simulink model "test_buildingblocks_newbasicblk_20150723"  (R2014a)
settings: Solver=ode45  StartTime=0.0  StopTime=100  FixedStep=0.001e-3  RelTol=1e-8  AbsTol=1e-11
values from neighbouring files (symbols this model uses):
  A_FB_EN = 1    [test_buildingblocks_newbasicblk_20150723_Sim.m]
  A_FB_EN0 = 1    [test_buildingblocks_newbasicblk_20150723_Sim.m]
  A_FB_EN01 = 0    [test_buildingblocks_newbasicblk_20150723_Sim.m]
  A_FB_EN1 = 1    [test_buildingblocks_newbasicblk_20150723_Sim.m]
  A_FB_EN12 = 0    [test_buildingblocks_newbasicblk_20150723_Sim.m]
  A_FB_EN4 = 0.5    [test_buildingblocks_newbasicblk_20150723_Sim.m]
  A_FB_EN5 = 0    [test_buildingblocks_newbasicblk_20150723_Sim.m]
  A_FB_EN_FI = 0    [test_buildingblocks_newbasicblk_20150723_Sim.m]
  B_FB_EN = 1    [test_buildingblocks_newbasicblk_20150723_Sim.m]
  B_FB_EN0 = 1    [test_buildingblocks_newbasicblk_20150723_Sim.m]
  B_FB_EN01 = 0    [test_buildingblocks_newbasicblk_20150723_Sim.m]
  B_FB_EN1 = 0    [test_buildingblocks_newbasicblk_20150723_Sim.m]
  B_FB_EN11 = 1    [test_buildingblocks_newbasicblk_20150723_Sim.m]
  B_FB_EN12 = 0    [test_buildingblocks_newbasicblk_20150723_Sim.m]
  B_FB_EN_FI = 0    [test_buildingblocks_newbasicblk_20150723_Sim.m]
  C_FF_EN = 1    [test_buildingblocks_newbasicblk_20150723_Sim.m]
  C_FF_ENb = 0    [test_buildingblocks_newbasicblk_20150723_Sim.m]
  D_FF_EN = 1    [test_buildingblocks_newbasicblk_20150723_Sim.m]
  D_FF_EN1 = 1    [test_buildingblocks_newbasicblk_20150723_Sim.m]
  KDfw = 10    [test_buildingblocks_newbasicblk_20150723_Model.m]    (also in test_buildingblocks_newbasicblk_20150723_Sim.m)
  KDfw0 = 10    [test_buildingblocks_newbasicblk_20150723_Sim.m]
  KDfw01 = 5    [test_buildingblocks_newbasicblk_20150723_Model.m]    (also in test_buildingblocks_newbasicblk_20150723_Sim.m)
  KDfw02 = 10    [test_buildingblocks_newbasicblk_20150723_Model.m]    (also in test_buildingblocks_newbasicblk_20150723_Sim.m)
  KDfw03 = 30    [test_buildingblocks_newbasicblk_20150723_Model.m]    (also in test_buildingblocks_newbasicblk_20150723_Sim.m)
  KDfw2 = 10    [test_buildingblocks_newbasicblk_20150723_Sim.m]
  KDrv = 10    [test_buildingblocks_newbasicblk_20150723_Model.m]    (also in test_buildingblocks_newbasicblk_20150723_Sim.m)
  KDrv0 = 10    [test_buildingblocks_newbasicblk_20150723_Sim.m]
  KDrv01 = 10    [test_buildingblocks_newbasicblk_20150723_Model.m]    (also in test_buildingblocks_newbasicblk_20150723_Sim.m)
  KDrv02 = 5    [test_buildingblocks_newbasicblk_20150723_Model.m]    (also in test_buildingblocks_newbasicblk_20150723_Sim.m)
  KDrv03 = 10    [test_buildingblocks_newbasicblk_20150723_Model.m]    (also in test_buildingblocks_newbasicblk_20150723_Sim.m)
  KDrv2 = 10    [test_buildingblocks_newbasicblk_20150723_Sim.m]
  KDrv5 = 10000000    [test_buildingblocks_newbasicblk_20150723_Sim.m]
  KDrv6 = 10000000    [test_buildingblocks_newbasicblk_20150723_Sim.m]
  kr1 = 10*kr_1/KDrv01    (= 10)    [test_buildingblocks_newbasicblk_20150723_Model.m]    (also in test_buildingblocks_newbasicblk_20150723_Sim.m)
  kr11 = 10    [test_buildingblocks_newbasicblk_20150723_Sim.m]
  kr1_01 = 5    [test_buildingblocks_newbasicblk_20150723_Sim.m]
  kr2 = 10*kr_1/KDrv02    (= 20)    [test_buildingblocks_newbasicblk_20150723_Model.m]    (also in test_buildingblocks_newbasicblk_20150723_Sim.m = 5)
  kr22 = 5    [test_buildingblocks_newbasicblk_20150723_Sim.m]
  krC = 10    [test_buildingblocks_newbasicblk_20150723_Sim.m]
  krC4 = 20    [test_buildingblocks_newbasicblk_20150723_Sim.m]
  krD = 10    [test_buildingblocks_newbasicblk_20150723_Sim.m]
  n = 1    [test_buildingblocks_newbasicblk_20150723_Sim.m]
  ratC = 0    [test_buildingblocks_newbasicblk_20150723_Sim.m]
  ratC0 = 0    [test_buildingblocks_newbasicblk_20150723_Sim.m]
  ratC01 = 1    [test_buildingblocks_newbasicblk_20150723_Sim.m]
  ratC02 = 0.1    [test_buildingblocks_newbasicblk_20150723_Sim.m]
  ratC03 = 2    [test_buildingblocks_newbasicblk_20150723_Sim.m]
  ratC04 = 0.5    [test_buildingblocks_newbasicblk_20150723_Sim.m]
  ratC05 = 10    [test_buildingblocks_newbasicblk_20150723_Sim.m]
  ratC10 = 0.06    [test_buildingblocks_newbasicblk_20150723_Model.m]    (also in test_buildingblocks_newbasicblk_20150723_Sim.m = 0.6)
  ratC11 = 0.2    [test_buildingblocks_newbasicblk_20150723_Sim.m]
  ratC12 = 0.2    [test_buildingblocks_newbasicblk_20150723_Model.m]    (also in test_buildingblocks_newbasicblk_20150723_Sim.m = 1)
  ratC13 = 0.2    [test_buildingblocks_newbasicblk_20150723_Model.m]    (also in test_buildingblocks_newbasicblk_20150723_Sim.m = 2)
  ratC14 = 0.3    [test_buildingblocks_newbasicblk_20150723_Model.m]    (also in test_buildingblocks_newbasicblk_20150723_Sim.m = 3)
  ratC15 = 0.2    [test_buildingblocks_newbasicblk_20150723_Model.m]    (also in test_buildingblocks_newbasicblk_20150723_Sim.m = 10)
  ratC4 = 1    [test_buildingblocks_newbasicblk_20150723_Model.m]    (also in test_buildingblocks_newbasicblk_20150723_Sim.m)
  ratC5 = 3    [test_buildingblocks_newbasicblk_20150723_Model.m]    (also in test_buildingblocks_newbasicblk_20150723_Sim.m)
  ratC7 = 1    [test_buildingblocks_newbasicblk_20150723_Model.m]    (also in test_buildingblocks_newbasicblk_20150723_Sim.m = 2)
  ratC8 = 0.1    [test_buildingblocks_newbasicblk_20150723_Model.m]    (also in test_buildingblocks_newbasicblk_20150723_Sim.m)
  ratC9 = 0.03    [test_buildingblocks_newbasicblk_20150723_Model.m]    (also in test_buildingblocks_newbasicblk_20150723_Sim.m = 0)
  ratD = 0    [test_buildingblocks_newbasicblk_20150723_Sim.m]
(part 1 of 3)
settings Model: Creator=lorenzo  LastModifiedBy=Sung
settings SolverCC: ZeroCrossControl=DisableAll
settings DataIOCC: SignalLoggingSaveFormat=ModelDataLogs
settings OptimizationCC: ExpressionDepthLimit=2147483647
settings DebuggingCC: UnderspecifiedInitializationDetection=Classic  FcnCallInpInsideContextMsg=UseLocalSettings  StateNameClashWarn=warning
settings GRTTargetCC: CombineOutputUpdateFcns=off  GRTInterface=on

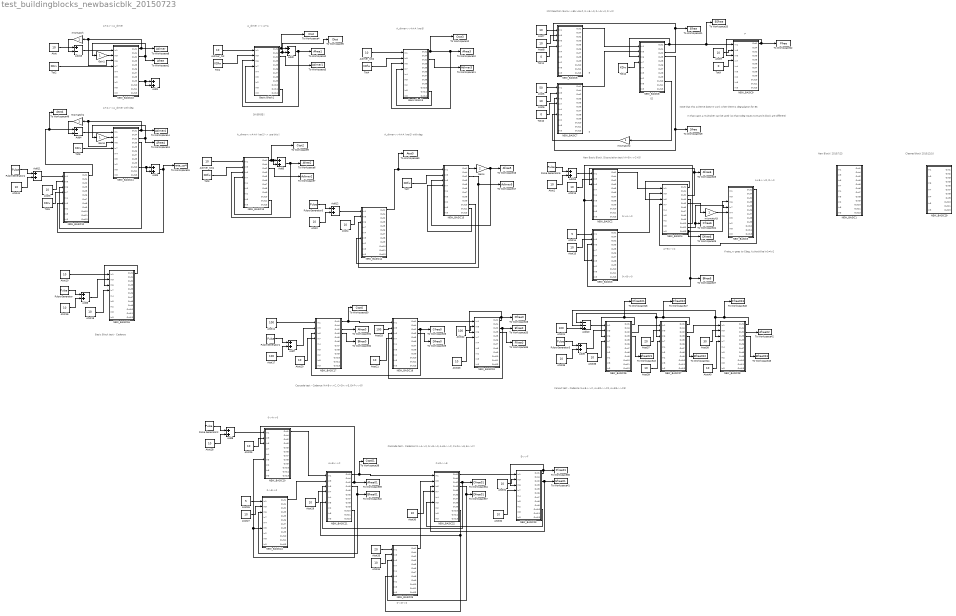
== system test_buildingblocks_newbasicblk_20150723 ==
  note: A+A<->A_dimer
  note: A_dimer <-> A+A
  note: DIVERGE!!
  note: A_dimer<->A+A (ver2) -> use this!!
  note: A_dimer<->A+A (ver3)
  note: A+A<->A_dimer with deg
  note: A_dimer<->A+A (ver2) with deg
  note: MM Reaction (E+S<->ES->E+P, 0->E->0, 0->S->0, P->0)
  note: P
  note: E
  note: S
  note: ES
  note: New Basic Block. Dissociation test (A+B<->C+D)
  note: A+B<->D, D->0
  note: A+B<->C
  note: 0->A->0
  note: 0->B->0
  note: New Block! 2015/7/23
  note: If rate_rv goes to Cdeg, it should be kr1=kr2
  note: Note that this scheme doesn't work when there is degradation for ES
  note: In that case, a multiplier can be used (so that Cdeg inputs to E and S block are different)
  note: Basic Block test - Cadence
  note: Cascade test - Cadence (A+B<->C, C+D<->E, E+F<->G)
  note: Cascade test - Cadence (0->A->0, 0->B->0, A+B<->C, C+D<->E, E<->F)
  note: 0->A->0
  note: A+B<->C
  note: 0->B->0
  note: C+D<->E
  note: E<->F
  note: 0->D->0
  note: Fanout test - Cadence (A+B<->C, A+B2<->C2, A+B3<->C3)
  note: Cleaned block 2015/12/10
  Add{1..3,5..9,11..13} (11 alike) : Sum
  Add10 : Sum  Inputs=--+
  Add15 : Sum  Inputs=+-
  Add4 : Sum  Inputs=+-
  Adimer_tot : Constant  Value=10
  Adimer_tot1 : Constant  Value=10
  Adimer_tot2 : Constant  Value=10
  Atot{,1..4,6..10,13,15..16,19..21,23,25,27..32,34..36,39..41} (30 alike) : Constant  Value=10
  Atot{11,17..18,22,24} (5 alike) : Constant  Value=100
  Atot14 : Constant  Value=5
  Atot26 : Constant  Value=5
  Atot33 : Constant  Value=20
  Atot37 : Constant  Value=20
  Atot38 : Constant  Value=30
  Atot5 : Constant  Value=50
  Basic Block1 : Subsystem
  Basic Block3 : Subsystem
  Gain1 : Gain
  Gain3 : Gain
  Gain4 : Gain  Gain=2
  NEW_BASIC1 : Subsystem
  NEW_BASIC10 : Subsystem
  NEW_BASIC11 : Subsystem
  NEW_BASIC12 : Subsystem
  NEW_BASIC13 : Subsystem
  NEW_BASIC14 : Subsystem
  NEW_BASIC15 : Subsystem
  NEW_BASIC16 : Subsystem
  NEW_BASIC17 : Subsystem
  NEW_BASIC18 : Subsystem
  NEW_BASIC19 : Subsystem
  NEW_BASIC2 : Subsystem
  NEW_BASIC20 : Subsystem
  NEW_BASIC21 : Subsystem
  NEW_BASIC22 : Subsystem
  NEW_BASIC23 : Subsystem
  NEW_BASIC24 : Subsystem
  NEW_BASIC25 : Subsystem
  NEW_BASIC26 : Subsystem
  NEW_BASIC27 : Subsystem
  NEW_BASIC28 : Subsystem
  NEW_BASIC29 : Subsystem
  NEW_BASIC3 : Subsystem
  NEW_BASIC4 : Subsystem
  NEW_BASIC5 : Subsystem
  NEW_BASIC6 : Subsystem
  NEW_BASIC7 : Subsystem
  NEW_BASIC8 : Subsystem
  NEW_BASIC9 : Subsystem
  Pulse Generator{,2..3,6} (4 alike) : DiscretePulseGenerator  PulseType=Time based  Amplitude=10  PulseWidth=50
  Pulse Generator1 : DiscretePulseGenerator  PulseType=Time based  Amplitude=100  PulseWidth=50
  Pulse Generator4 : DiscretePulseGenerator  PulseType=Time based  Amplitude=10  Period=4  PulseWidth=50
  Pulse Generator5 : DiscretePulseGenerator  PulseType=Time based  Amplitude=10  Period=4  PulseWidth=50
  To Workspace1 : ToWorkspace  VariableName=Afree  SaveFormat=Timeseries  SampleTime=-1
  To Workspace10 : ToWorkspace  VariableName=Afree3  SaveFormat=Timeseries  SampleTime=-1
  To Workspace11 : ToWorkspace  VariableName=Adimer3  SaveFormat=Timeseries  SampleTime=-1
  To Workspace12 : ToWorkspace  VariableName=Ctot3  SaveFormat=Timeseries  SampleTime=-1
  To Workspace13 : ToWorkspace  VariableName=Afree4  SaveFormat=Timeseries  SampleTime=-1
  To Workspace14 : ToWorkspace  VariableName=Adimer4  SaveFormat=Timeseries  SampleTime=-1
  To Workspace15 : ToWorkspace  VariableName=rate_up4  SaveFormat=Timeseries  SampleTime=-1
  To Workspace16 : ToWorkspace  VariableName=Afree5  SaveFormat=Timeseries  SampleTime=-1
  To Workspace17 : ToWorkspace  VariableName=Adimer5  SaveFormat=Timeseries  SampleTime=-1
  To Workspace19 : ToWorkspace  VariableName=Sfree  SaveFormat=Timeseries  SampleTime=-1
  To Workspace2 : ToWorkspace  VariableName=Afree1  SaveFormat=Timeseries  SampleTime=-1
  To Workspace20 : ToWorkspace  VariableName=ESfree  SaveFormat=Timeseries  SampleTime=-1
  To Workspace21 : ToWorkspace  VariableName=Efree  SaveFormat=Timeseries  SampleTime=-1
  To Workspace22 : ToWorkspace  VariableName=Pfree  SaveFormat=Timeseries  SampleTime=-1
  To Workspace23 : ToWorkspace  VariableName=Afree6  SaveFormat=Timeseries  SampleTime=-1
  To Workspace24 : ToWorkspace  VariableName=Cfree6  SaveFormat=Timeseries  SampleTime=-1
  To Workspace25 : ToWorkspace  VariableName=Dfree6  SaveFormat=Timeseries  SampleTime=-1
  To Workspace26 : ToWorkspace  VariableName=Cfree0  SaveFormat=Timeseries  SampleTime=-1
  To Workspace27 : ToWorkspace  VariableName=Bfree6  SaveFormat=Timeseries  SampleTime=-1
  To Workspace28 : ToWorkspace  VariableName=Gfree0  SaveFormat=Timeseries  SampleTime=-1
  To Workspace29 : ToWorkspace  VariableName=Dfree0  SaveFormat=Timeseries  SampleTime=-1
  To Workspace3 : ToWorkspace  VariableName=Adimer1  SaveFormat=Timeseries  SampleTime=-1
  To Workspace30 : ToWorkspace  VariableName=Ctot0  SaveFormat=Timeseries  SampleTime=-1
  To Workspace31 : ToWorkspace  VariableName=Afree0  SaveFormat=Timeseries  SampleTime=-1
  To Workspace32 : ToWorkspace  VariableName=Bfree0  SaveFormat=Timeseries  SampleTime=-1
  To Workspace33 : ToWorkspace  VariableName=Efree0  SaveFormat=Timeseries  SampleTime=-1
  To Workspace34 : ToWorkspace  VariableName=Cfree01  SaveFormat=Timeseries  SampleTime=-1
  To Workspace35 : ToWorkspace  VariableName=Ffree0  SaveFormat=Timeseries  SampleTime=-1
  To Workspace36 : ToWorkspace  VariableName=Ffree01  SaveFormat=Timeseries  SampleTime=-1
  To Workspace37 : ToWorkspace  VariableName=Dfree01  SaveFormat=Timeseries  SampleTime=-1
  To Workspace38 : ToWorkspace  VariableName=Ctot01  SaveFormat=Timeseries  SampleTime=-1
  To Workspace39 : ToWorkspace  VariableName=Afree01  SaveFormat=Timeseries  SampleTime=-1
  To Workspace4 : ToWorkspace  VariableName=Ctot  SaveFormat=Timeseries  SampleTime=-1
  To Workspace40 : ToWorkspace  VariableName=Bfree01  SaveFormat=Timeseries  SampleTime=-1
  To Workspace41 : ToWorkspace  VariableName=Efree01  SaveFormat=Timeseries  SampleTime=-1
  To Workspace42 : ToWorkspace  VariableName=Afree02  SaveFormat=Timeseries  SampleTime=-1
  To Workspace43 : ToWorkspace  VariableName=Bfree021  SaveFormat=Timeseries  SampleTime=-1
  To Workspace44 : ToWorkspace  VariableName=Bfree022  SaveFormat=Timeseries  SampleTime=-1
  To Workspace45 : ToWorkspace  VariableName=Bfree023  SaveFormat=Timeseries  SampleTime=-1
  To Workspace46 : ToWorkspace  VariableName=Cfree021  SaveFormat=Timeseries  SampleTime=-1
  To Workspace47 : ToWorkspace  VariableName=Cfree022  SaveFormat=Timeseries  SampleTime=-1
  To Workspace48 : ToWorkspace  VariableName=Cfree023  SaveFormat=Timeseries  SampleTime=-1
  To Workspace49 : ToWorkspace  VariableName=Atot4  SaveFormat=Timeseries  SampleTime=-1
  To Workspace5 : ToWorkspace  VariableName=Dtot  SaveFormat=Timeseries  SampleTime=-1
  To Workspace50 : ToWorkspace  VariableName=Atot5  SaveFormat=Timeseries  SampleTime=-1
  To Workspace6 : ToWorkspace  VariableName=Afree2  SaveFormat=Timeseries  SampleTime=-1
  To Workspace7 : ToWorkspace  VariableName=Adimer2  SaveFormat=Timeseries  SampleTime=-1
  To Workspace8 : ToWorkspace  VariableName=Adimer  SaveFormat=Timeseries  SampleTime=-1
  To Workspace9 : ToWorkspace  VariableName=Ctot2  SaveFormat=Timeseries  SampleTime=-1
  Tot{1,3..4,7} (4 alike) : Constant  Value=KDfw
  Tot10 : Constant  Value=0
  Tot11 : Constant  Value=0
  Tot{2,5..6,12} (4 alike) : Constant  Value=KDrv
  Tot9 : Constant  Value=0
  mismatch{,1..3} (4 alike) : Gain
  wires:
  Add15/1 -> NEW_BASIC10/1(In1)
  Atot/1 -> Add15/1
  NEW_BASIC10/1(Out1) -> To Workspace8/1, NEW_BASIC10/3(In6), mismatch/1
  NEW_BASIC10/3(Out2) -> To Workspace1/1, Gain1/1
  Tot2/1 -> NEW_BASIC10/4(In7)
  Adimer_tot/1 -> Basic Block1/1(In1)
  Basic Block1/11(Out11) -> Basic Block1/4(In7)
  Tot1/1 -> Basic Block1/2(In9)
  Basic Block1/1(Out1) -> To Workspace4/1, Add2/1
  Basic Block1/2(Out4) -> To Workspace5/1, Add2/2
  Add2/1 -> To Workspace2/1, Basic Block1/3(In6)
  Basic Block1/3(Out2) -> To Workspace3/1
  Adimer_tot1/1 -> NEW_BASIC13/1(In1)
  Tot3/1 -> NEW_BASIC13/2(In9)
  NEW_BASIC13/1(Out1) -> Add5/2, Add5/1, To Workspace9/1
  Add5/1 -> NEW_BASIC13/3(In6), To Workspace6/1
  NEW_BASIC13/3(Out2) -> To Workspace7/1
  NEW_BASIC13/11(Out11) -> NEW_BASIC13/4(In7)
  Adimer_tot2/1 -> Basic Block3/1(In1)
  Tot4/1 -> Basic Block3/2(In9)
  Basic Block3/1(Out1) -> Basic Block3/3(In6), To Workspace10/1, To Workspace12/1
  Basic Block3/3(Out2) -> To Workspace11/1
  Basic Block3/11(Out11) -> Basic Block3/4(In7)
  mismatch/1 -> Add15/2
  Gain1/1 -> NEW_BASIC10/2(In9)
  NEW_BASIC10/9(Out9) -> Add1/2, Add1/1
  Add4/1 -> NEW_BASIC11/1(In1)
  NEW_BASIC12/1(Out1) -> To Workspace49/1, Add4/1
  NEW_BASIC11/1(Out1) -> NEW_BASIC11/3(In6), mismatch1/1, To Workspace14/1
  NEW_BASIC11/3(Out2) -> Gain3/1, To Workspace13/1
  Tot5/1 -> NEW_BASIC11/4(In7)
  mismatch1/1 -> Add4/2
  Gain3/1 -> NEW_BASIC11/2(In9)
  Add11/1 -> NEW_BASIC12/1(In1)
  Atot3/1 -> NEW_BASIC12/2(In9)
  Tot6/1 -> NEW_BASIC12/4(In7)
  NEW_BASIC11/4(Out3) -> NEW_BASIC12/3(In6)
  Add3/1 -> NEW_BASIC12/6(In5), To Workspace15/1
  NEW_BASIC11/10(Out10) -> Add3/2, Add3/1
  NEW_BASIC14/1(Out1) -> To Workspace50/1, NEW_BASIC15/1(In1)
  Tot7/1 -> NEW_BASIC15/2(In9)
  NEW_BASIC15/1(Out1) -> Gain4/1
  Gain4/1 -> NEW_BASIC15/3(In6), To Workspace16/1
  NEW_BASIC15/3(Out2) -> NEW_BASIC14/3(In6), To Workspace17/1
  NEW_BASIC15/11(Out11) -> NEW_BASIC15/4(In7)
  Atot4/1 -> NEW_BASIC14/2(In9)
  NEW_BASIC15/10(Out10) -> NEW_BASIC14/6(In5)
  Atot5/1 -> NEW_BASIC7/1(In1)
  Atot6/1 -> NEW_BASIC7/2(In9)
  Tot10/1 -> NEW_BASIC7/4(In7)
  NEW_BASIC8/10(Out10) -> mismatch2/1
  Atot7/1 -> NEW_BASIC6/1(In1)
  Atot8/1 -> NEW_BASIC6/2(In9)
  Tot11/1 -> NEW_BASIC6/4(In7)
  NEW_BASIC6/1(Out1) -> NEW_BASIC8/1(In1)
  NEW_BASIC7/1(Out1) -> NEW_BASIC8/2(In9)
  NEW_BASIC8/3(Out2) -> NEW_BASIC6/3(In6), To Workspace21/1
  NEW_BASIC8/4(Out3) -> NEW_BASIC7/3(In6), To Workspace19/1
  NEW_BASIC8/1(Out1) -> NEW_BASIC8/3(In6), NEW_BASIC9/1(In1), To Workspace20/1
  Atot9/1 -> NEW_BASIC9/2(In9)
  Tot9/1 -> NEW_BASIC9/4(In7)
  NEW_BASIC9/1(Out1) -> NEW_BASIC9/3(In6), To Workspace22/1
  Tot12/1 -> NEW_BASIC8/4(In7)
  mismatch2/1 -> NEW_BASIC7/6(In5)
  NEW_BASIC4/5(Out5) -> mismatch3/1
  NEW_BASIC4/1(Out1) -> NEW_BASIC4/3(In6)
  NEW_BASIC5/1(Out1) -> NEW_BASIC4/4(In7)
  NEW_BASIC4/11(Out11) -> NEW_BASIC5/4(In7), To Workspace24/1
  NEW_BASIC4/12(Out13) -> NEW_BASIC5/3(In6), To Workspace25/1
  NEW_BASIC4/4(Out3) -> NEW_BASIC3/3(In6), To Workspace27/1
  mismatch3/1 -> NEW_BASIC5/5(In4)
  Atot13/1 -> NEW_BASIC2/2(In9)
  Atot14/1 -> NEW_BASIC3/1(In1)
  Atot15/1 -> NEW_BASIC3/2(In9)
  NEW_BASIC2/1(Out1) -> NEW_BASIC4/1(In1)
  NEW_BASIC3/1(Out1) -> NEW_BASIC4/2(In9)
  NEW_BASIC4/3(Out2) -> NEW_BASIC2/3(In6), To Workspace23/1
  NEW_BASIC4/10(Out10) -> NEW_BASIC3/6(In5), NEW_BASIC2/6(In5)
  Atot10/1 -> NEW_BASIC16/1(In1)
  NEW_BASIC16/1(Out1) -> NEW_BASIC16/3(In6)
  Pulse Generator/1 -> Add6/1
  Atot16/1 -> Add6/2
  Add6/1 -> NEW_BASIC16/2(In9)
  Atot11/1 -> NEW_BASIC17/1(In1)
  Pulse Generator1/1 -> Add7/1
  Atot17/1 -> Add7/2
  Add7/1 -> NEW_BASIC17/2(In9)
  NEW_BASIC17/1(Out1) -> To Workspace30/1, NEW_BASIC18/1(In1)
  Atot18/1 -> NEW_BASIC18/2(In9)
  NEW_BASIC18/3(Out2) -> To Workspace26/1, NEW_BASIC17/3(In6)
  Atot19/1 -> NEW_BASIC16/4(In7)
  Atot20/1 -> NEW_BASIC17/4(In7)
  Atot21/1 -> NEW_BASIC18/4(In7)
  NEW_BASIC17/3(Out2) -> To Workspace31/1
  NEW_BASIC17/4(Out3) -> To Workspace32/1
  NEW_BASIC18/4(Out3) -> To Workspace29/1
  Atot22/1 -> NEW_BASIC19/2(In9)
  Atot23/1 -> NEW_BASIC19/4(In7)
  NEW_BASIC19/4(Out3) -> To Workspace35/1
  NEW_BASIC18/1(Out1) -> NEW_BASIC19/1(In1)
  NEW_BASIC19/1(Out1) -> To Workspace28/1, NEW_BASIC19/3(In6)
  NEW_BASIC19/3(Out2) -> NEW_BASIC18/3(In6), To Workspace33/1
  Add8/1 -> NEW_BASIC20/1(In1)
  Atot25/1 -> NEW_BASIC20/2(In9)
  NEW_BASIC21/1(Out1) -> NEW_BASIC22/1(In1), To Workspace38/1
  NEW_BASIC22/3(Out2) -> NEW_BASIC21/3(In6), To Workspace34/1
  Atot29/1 -> NEW_BASIC21/4(In7)
  Atot30/1 -> NEW_BASIC22/4(In7)
  NEW_BASIC21/3(Out2) -> NEW_BASIC20/3(In6), To Workspace39/1
  NEW_BASIC21/4(Out3) -> NEW_BASIC24/3(In6), To Workspace40/1
  NEW_BASIC22/4(Out3) -> NEW_BASIC25/3(In6), To Workspace37/1
  Atot31/1 -> NEW_BASIC23/2(In9)
  Atot32/1 -> NEW_BASIC23/4(In7)
  NEW_BASIC22/1(Out1) -> NEW_BASIC23/1(In1)
  NEW_BASIC23/1(Out1) -> NEW_BASIC23/3(In6), To Workspace36/1
  NEW_BASIC23/3(Out2) -> To Workspace41/1, NEW_BASIC22/3(In6)
  Atot26/1 -> NEW_BASIC24/1(In1)
  Atot27/1 -> NEW_BASIC24/2(In9)
  NEW_BASIC20/1(Out1) -> NEW_BASIC21/1(In1)
  NEW_BASIC24/1(Out1) -> NEW_BASIC21/2(In9)
  Atot33/1 -> NEW_BASIC25/1(In1)
  Atot34/1 -> NEW_BASIC25/2(In9)
  NEW_BASIC25/1(Out1) -> NEW_BASIC22/2(In9)
  NEW_BASIC23/10(Out10) -> NEW_BASIC22/6(In5)
  NEW_BASIC22/10(Out10) -> NEW_BASIC25/6(In5), NEW_BASIC21/6(In5)
  NEW_BASIC21/10(Out10) -> NEW_BASIC24/6(In5), NEW_BASIC20/6(In5)
  Pulse Generator2/1 -> Add8/1
  Atot28/1 -> Add8/2
  Pulse Generator3/1 -> Add9/1
  Atot35/1 -> Add9/2
  Add9/1 -> NEW_BASIC26/2(In9)
  NEW_BASIC26/1(Out1) -> To Workspace46/1, NEW_BASIC26/3(In6)
  Add10/1 -> NEW_BASIC26/1(In1)
  Atot24/1 -> Add10/3
  NEW_BASIC27/1(Out1) -> To Workspace47/1, Add10/1, NEW_BASIC27/3(In6)
  NEW_BASIC28/1(Out1) -> To Workspace48/1, NEW_BASIC28/3(In6), Add10/2
  NEW_BASIC26/3(Out2) -> NEW_BASIC27/1(In1)
  NEW_BASIC27/3(Out2) -> NEW_BASIC28/1(In1)
  NEW_BASIC28/3(Out2) -> To Workspace42/1
  Atot37/1 -> NEW_BASIC27/2(In9)
  Atot38/1 -> NEW_BASIC28/2(In9)
  NEW_BASIC26/4(Out3) -> To Workspace43/1
  NEW_BASIC28/4(Out3) -> To Workspace45/1
  NEW_BASIC27/4(Out3) -> To Workspace44/1
  Atot36/1 -> NEW_BASIC26/4(In7)
  Atot39/1 -> NEW_BASIC27/4(In7)
  Atot40/1 -> NEW_BASIC28/4(In7)
  Pulse Generator4/1 -> Add11/1
  Atot41/1 -> Add11/2
  Pulse Generator5/1 -> Add12/1
  Atot2/1 -> Add12/2
  Add12/1 -> NEW_BASIC14/1(In1)
  Pulse Generator6/1 -> Add13/1
  Atot1/1 -> Add13/2
  Add13/1 -> NEW_BASIC2/1(In1)

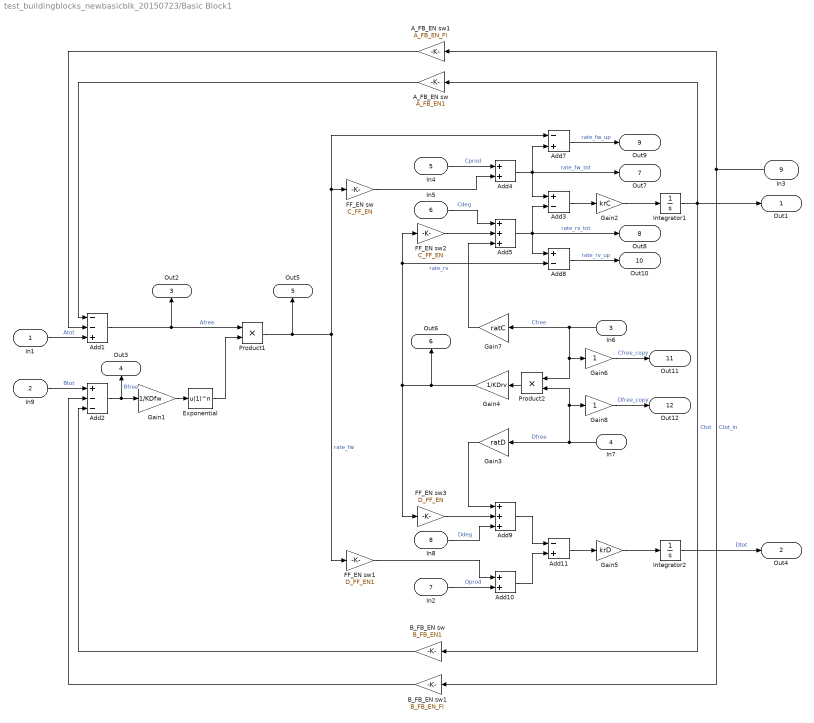
== system test_buildingblocks_newbasicblk_20150723/Basic Block1 ==
  In1 : Inport
  In9 : Inport  Port=2
  In6 : Inport  Port=3
  In7 : Inport  Port=4
  In4 : Inport  Port=5
  In5 : Inport  Port=6
  In2 : Inport  Port=7
  In8 : Inport  Port=8
  In3 : Inport  Port=9
  A_FB_EN sw : Gain  Gain=A_FB_EN1
  A_FB_EN sw1 : Gain  Gain=A_FB_EN_FI
  Add1 : Sum  Inputs=--+
  Add10 : Sum
  Add11 : Sum  Inputs=-+
  Add2 : Sum  Inputs=+--
  Add3 : Sum  Inputs=+-
  Add4 : Sum
  Add5 : Sum  Inputs=+++
  Add7 : Sum  Inputs=-+
  Add8 : Sum  Inputs=+-
  Add9 : Sum  Inputs=+++
  B_FB_EN sw : Gain  Gain=B_FB_EN1
  B_FB_EN sw1 : Gain  Gain=B_FB_EN_FI
  Exponential : Fcn  Expr=u(1)^n
  FF_EN sw : Gain  Gain=C_FF_EN
  FF_EN sw1 : Gain  Gain=D_FF_EN1
  FF_EN sw2 : Gain  Gain=C_FF_EN
  FF_EN sw3 : Gain  Gain=D_FF_EN
  Gain1 : Gain  Gain=1/KDfw
  Gain2 : Gain  Gain=krC
  Gain3 : Gain  Gain=ratD
  Gain4 : Gain  Gain=1/KDrv
  Gain5 : Gain  Gain=krD
  Gain6 : Gain
  Gain7 : Gain  Gain=ratC
  Gain8 : Gain
  Integrator1 : Integrator
  Integrator2 : Integrator
  Product1 : Product  RndMeth=Zero
  Product2 : Product  RndMeth=Zero
  Out1 : Outport
  Out4 : Outport  Port=2
  Out2 : Outport  Port=3
  Out3 : Outport  Port=4
  Out5 : Outport  Port=5
  Out6 : Outport  Port=6
  Out7 : Outport  Port=7
  Out8 : Outport  Port=8
  Out9 : Outport  Port=9
  Out10 : Outport  Port=10
  Out11 : Outport  Port=11
  Out12 : Outport  Port=12
  wires:
  B_FB_EN sw/1 -> Add2/3
  A_FB_EN sw/1 -> Add1/1
  Add3/1 -> Gain2/1
  Add2/1 -> Gain1/1, Out3/1  "Bfree"
  Add1/1 -> Out2/1, Product1/1  "Afree"
  In1/1 -> Add1/3  "Atot"
  In9/1 -> Add2/1  "Btot"
  Gain1/1 -> Exponential/1
  Exponential/1 -> Product1/2
  Integrator1/1 -> B_FB_EN sw/1, Out1/1, A_FB_EN sw/1  "Ctot"
  Gain2/1 -> Integrator1/1
  In6/1 -> Gain6/1, Product2/1, Gain7/1  "Cfree"
  In7/1 -> Gain3/1, Gain8/1, Product2/2  "Dfree"
  Product2/1 -> Gain4/1
  Gain5/1 -> Integrator2/1
  Integrator2/1 -> Out4/1  "Dtot"
  Gain4/1 -> Out6/1, Add8/2, FF_EN sw2/1, FF_EN sw3/1  "rate_rv"
  Product1/1 -> Out5/1, FF_EN sw1/1, Add7/1, FF_EN sw/1  "rate_fw"
  FF_EN sw1/1 -> Add10/1
  In8/1 -> Add9/3  "Ddeg"
  In4/1 -> Add4/1  "Cprod"
  In5/1 -> Add5/1  "Cdeg"
  Gain7/1 -> Add5/3
  Gain3/1 -> Add9/1
  In3/1 -> B_FB_EN sw1/1, A_FB_EN sw1/1  "Ctot_in"
  A_FB_EN sw1/1 -> Add1/2
  B_FB_EN sw1/1 -> Add2/2
  Add4/1 -> Add7/2, Out7/1, Add3/1  "rate_fw_tot"
  Add5/1 -> Add8/1, Out8/1, Add3/2  "rate_rv_tot"
  FF_EN sw/1 -> Add4/2
  Add7/1 -> Out9/1  "rate_fw_up"
  Add8/1 -> Out10/1  "rate_rv_up"
  Gain6/1 -> Out11/1  "Cfree_copy"
  Gain8/1 -> Out12/1  "Dfree_copy"
  In2/1 -> Add10/2  "Dprod"
  Add9/1 -> Add11/1
  Add10/1 -> Add11/2
  Add11/1 -> Gain5/1
  FF_EN sw2/1 -> Add5/2
  FF_EN sw3/1 -> Add9/2

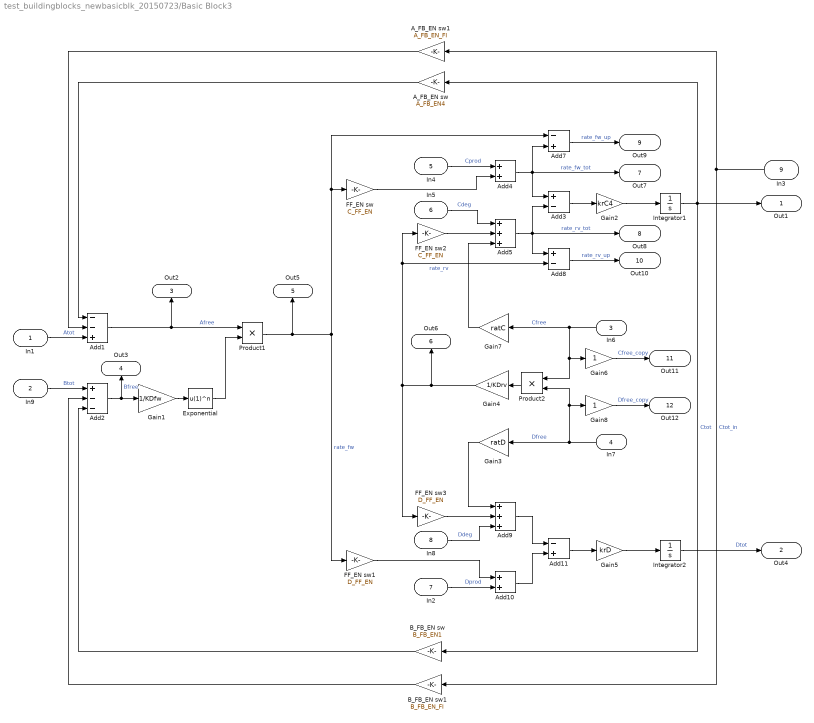
== system test_buildingblocks_newbasicblk_20150723/Basic Block3 ==
  In1 : Inport
  In9 : Inport  Port=2
  In6 : Inport  Port=3
  In7 : Inport  Port=4
  In4 : Inport  Port=5
  In5 : Inport  Port=6
  In2 : Inport  Port=7
  In8 : Inport  Port=8
  In3 : Inport  Port=9
  A_FB_EN sw : Gain  Gain=A_FB_EN4
  A_FB_EN sw1 : Gain  Gain=A_FB_EN_FI
  Add1 : Sum  Inputs=--+
  Add10 : Sum
  Add11 : Sum  Inputs=-+
  Add2 : Sum  Inputs=+--
  Add3 : Sum  Inputs=+-
  Add4 : Sum
  Add5 : Sum  Inputs=+++
  Add7 : Sum  Inputs=-+
  Add8 : Sum  Inputs=+-
  Add9 : Sum  Inputs=+++
  B_FB_EN sw : Gain  Gain=B_FB_EN1
  B_FB_EN sw1 : Gain  Gain=B_FB_EN_FI
  Exponential : Fcn  Expr=u(1)^n
  FF_EN sw : Gain  Gain=C_FF_EN
  FF_EN sw1 : Gain  Gain=D_FF_EN
  FF_EN sw2 : Gain  Gain=C_FF_EN
  FF_EN sw3 : Gain  Gain=D_FF_EN
  Gain1 : Gain  Gain=1/KDfw
  Gain2 : Gain  Gain=krC4
  Gain3 : Gain  Gain=ratD
  Gain4 : Gain  Gain=1/KDrv
  Gain5 : Gain  Gain=krD
  Gain6 : Gain
  Gain7 : Gain  Gain=ratC
  Gain8 : Gain
  Integrator1 : Integrator
  Integrator2 : Integrator
  Product1 : Product  RndMeth=Zero
  Product2 : Product  RndMeth=Zero
  Out1 : Outport
  Out4 : Outport  Port=2
  Out2 : Outport  Port=3
  Out3 : Outport  Port=4
  Out5 : Outport  Port=5
  Out6 : Outport  Port=6
  Out7 : Outport  Port=7
  Out8 : Outport  Port=8
  Out9 : Outport  Port=9
  Out10 : Outport  Port=10
  Out11 : Outport  Port=11
  Out12 : Outport  Port=12
  wires:
  B_FB_EN sw/1 -> Add2/3
  A_FB_EN sw/1 -> Add1/1
  Add3/1 -> Gain2/1
  Add2/1 -> Gain1/1, Out3/1  "Bfree"
  Add1/1 -> Out2/1, Product1/1  "Afree"
  In1/1 -> Add1/3  "Atot"
  In9/1 -> Add2/1  "Btot"
  Gain1/1 -> Exponential/1
  Exponential/1 -> Product1/2
  Integrator1/1 -> B_FB_EN sw/1, Out1/1, A_FB_EN sw/1  "Ctot"
  Gain2/1 -> Integrator1/1
  In6/1 -> Gain6/1, Product2/1, Gain7/1  "Cfree"
  In7/1 -> Gain3/1, Gain8/1, Product2/2  "Dfree"
  Product2/1 -> Gain4/1
  Gain5/1 -> Integrator2/1
  Integrator2/1 -> Out4/1  "Dtot"
  Gain4/1 -> Out6/1, Add8/2, FF_EN sw2/1, FF_EN sw3/1  "rate_rv"
  Product1/1 -> Out5/1, FF_EN sw1/1, Add7/1, FF_EN sw/1  "rate_fw"
  FF_EN sw1/1 -> Add10/1
  In8/1 -> Add9/3  "Ddeg"
  In4/1 -> Add4/1  "Cprod"
  In5/1 -> Add5/1  "Cdeg"
  Gain7/1 -> Add5/3
  Gain3/1 -> Add9/1
  In3/1 -> B_FB_EN sw1/1, A_FB_EN sw1/1  "Ctot_in"
  A_FB_EN sw1/1 -> Add1/2
  B_FB_EN sw1/1 -> Add2/2
  Add4/1 -> Add7/2, Out7/1, Add3/1  "rate_fw_tot"
  Add5/1 -> Add8/1, Out8/1, Add3/2  "rate_rv_tot"
  FF_EN sw/1 -> Add4/2
  Add7/1 -> Out9/1  "rate_fw_up"
  Add8/1 -> Out10/1  "rate_rv_up"
  Gain6/1 -> Out11/1  "Cfree_copy"
  Gain8/1 -> Out12/1  "Dfree_copy"
  In2/1 -> Add10/2  "Dprod"
  Add9/1 -> Add11/1
  Add10/1 -> Add11/2
  Add11/1 -> Gain5/1
  FF_EN sw2/1 -> Add5/2
  FF_EN sw3/1 -> Add9/2

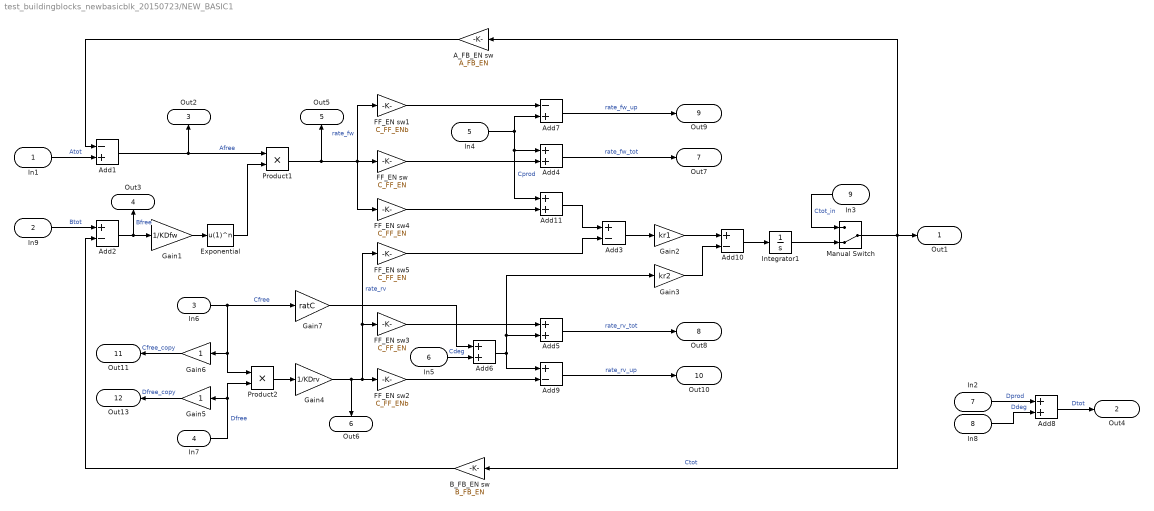
== system test_buildingblocks_newbasicblk_20150723/NEW_BASIC1 ==
  In1 : Inport
  In9 : Inport  Port=2
  In6 : Inport  Port=3
  In7 : Inport  Port=4
  In4 : Inport  Port=5
  In5 : Inport  Port=6
  In2 : Inport  Port=7
  In8 : Inport  Port=8
  In3 : Inport  Port=9
  A_FB_EN sw : Gain  Gain=A_FB_EN
  Add1 : Sum  Inputs=-+
  Add{2..3,9..10} (4 alike) : Sum  Inputs=+-
  Add{4..6,8,11} (5 alike) : Sum
  Add7 : Sum  Inputs=-+
  B_FB_EN sw : Gain  Gain=B_FB_EN
  Exponential : Fcn  Expr=u(1)^n
  FF_EN sw{,3..5} (4 alike) : Gain  Gain=C_FF_EN
  FF_EN sw1 : Gain  Gain=C_FF_ENb
  FF_EN sw2 : Gain  Gain=C_FF_ENb
  Gain1 : Gain  Gain=1/KDfw
  Gain2 : Gain  Gain=kr1
  Gain3 : Gain  Gain=kr2
  Gain4 : Gain  Gain=1/KDrv
  Gain5 : Gain
  Gain6 : Gain
  Gain7 : Gain  Gain=ratC
  Integrator1 : Integrator
  Manual Switch : ManualSwitch  CurrentSetting=0
  Product1 : Product  RndMeth=Zero
  Product2 : Product  RndMeth=Zero
  Out1 : Outport
  Out4 : Outport  Port=2
  Out2 : Outport  Port=3
  Out3 : Outport  Port=4
  Out5 : Outport  Port=5
  Out6 : Outport  Port=6
  Out7 : Outport  Port=7
  Out8 : Outport  Port=8
  Out9 : Outport  Port=9
  Out10 : Outport  Port=10
  Out11 : Outport  Port=11
  Out13 : Outport  Port=12
  wires:
  Gain5/1 -> Out13/1  "Dfree_copy"
  B_FB_EN sw/1 -> Add2/2
  A_FB_EN sw/1 -> Add1/1
  Add3/1 -> Gain2/1
  Add2/1 -> Gain1/1, Out3/1  "Bfree"
  Add1/1 -> Out2/1, Product1/1  "Afree"
  In1/1 -> Add1/2  "Atot"
  In9/1 -> Add2/1  "Btot"
  Gain1/1 -> Exponential/1
  Exponential/1 -> Product1/2
  Product1/1 -> Out5/1, FF_EN sw/1, FF_EN sw4/1, FF_EN sw1/1  "rate_fw"
  In4/1 -> Add11/1, Add4/1, Add7/2  "Cprod"
  Add4/1 -> Out7/1  "rate_fw_tot"
  FF_EN sw/1 -> Add4/2
  Add7/1 -> Out9/1  "rate_fw_up"
  Add9/1 -> Out10/1  "rate_rv_up"
  In3/1 -> Manual Switch/1  "Ctot_in"
  Integrator1/1 -> Manual Switch/2
  Manual Switch/1 -> B_FB_EN sw/1, A_FB_EN sw/1, Out1/1  "Ctot"
  FF_EN sw1/1 -> Add7/1
  In5/1 -> Add6/2  "Cdeg"
  In6/1 -> Gain6/1, Product2/1, Gain7/1  "Cfree"
  In7/1 -> Product2/2, Gain5/1  "Dfree"
  Product2/1 -> Gain4/1
  Gain6/1 -> Out11/1  "Cfree_copy"
  Gain4/1 -> FF_EN sw5/1, FF_EN sw3/1, FF_EN sw2/1, Out6/1  "rate_rv"
  FF_EN sw3/1 -> Add5/1
  FF_EN sw2/1 -> Add9/2
  Add6/1 -> Gain3/1, Add5/2, Add9/1
  Add5/1 -> Out8/1  "rate_rv_tot"
  Gain7/1 -> Add6/1
  In2/1 -> Add8/1  "Dprod"
  In8/1 -> Add8/2  "Ddeg"
  Add8/1 -> Out4/1  "Dtot"
  Add10/1 -> Integrator1/1
  Gain2/1 -> Add10/1
  Gain3/1 -> Add10/2
  Add11/1 -> Add3/1
  FF_EN sw4/1 -> Add11/2
  FF_EN sw5/1 -> Add3/2

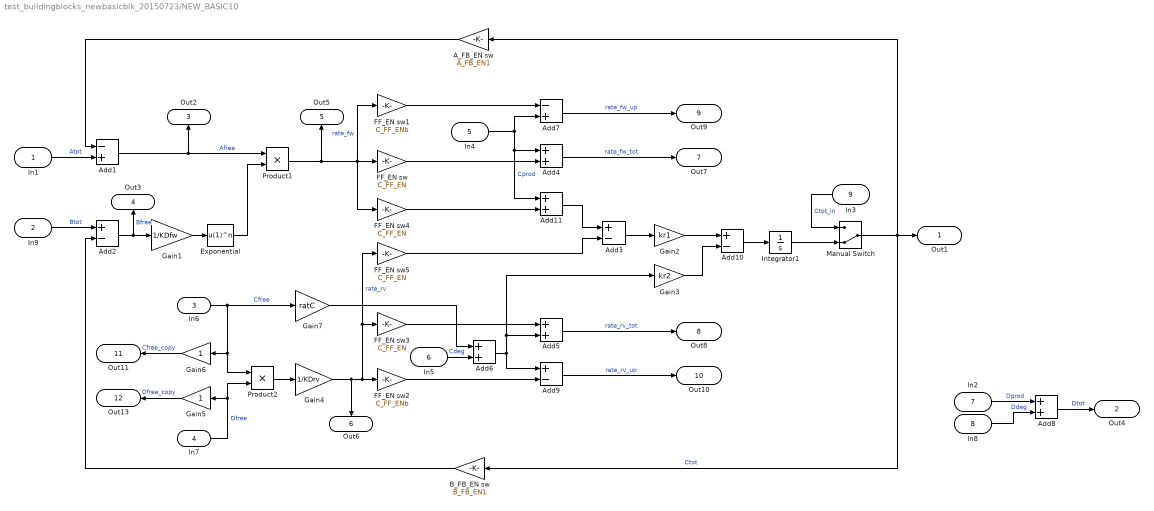
== system test_buildingblocks_newbasicblk_20150723/NEW_BASIC10 ==
  In1 : Inport
  In9 : Inport  Port=2
  In6 : Inport  Port=3
  In7 : Inport  Port=4
  In4 : Inport  Port=5
  In5 : Inport  Port=6
  In2 : Inport  Port=7
  In8 : Inport  Port=8
  In3 : Inport  Port=9
  A_FB_EN sw : Gain  Gain=A_FB_EN1
  Add1 : Sum  Inputs=-+
  Add{2..3,9..10} (4 alike) : Sum  Inputs=+-
  Add{4..6,8,11} (5 alike) : Sum
  Add7 : Sum  Inputs=-+
  B_FB_EN sw : Gain  Gain=B_FB_EN1
  Exponential : Fcn  Expr=u(1)^n
  FF_EN sw{,3..5} (4 alike) : Gain  Gain=C_FF_EN
  FF_EN sw1 : Gain  Gain=C_FF_ENb
  FF_EN sw2 : Gain  Gain=C_FF_ENb
  Gain1 : Gain  Gain=1/KDfw
  Gain2 : Gain  Gain=kr1
  Gain3 : Gain  Gain=kr2
  Gain4 : Gain  Gain=1/KDrv
  Gain5 : Gain
  Gain6 : Gain
  Gain7 : Gain  Gain=ratC
  Integrator1 : Integrator
  Manual Switch : ManualSwitch  CurrentSetting=0
  Product1 : Product  RndMeth=Zero
  Product2 : Product  RndMeth=Zero
  Out1 : Outport
  Out4 : Outport  Port=2
  Out2 : Outport  Port=3
  Out3 : Outport  Port=4
  Out5 : Outport  Port=5
  Out6 : Outport  Port=6
  Out7 : Outport  Port=7
  Out8 : Outport  Port=8
  Out9 : Outport  Port=9
  Out10 : Outport  Port=10
  Out11 : Outport  Port=11
  Out13 : Outport  Port=12
  wires:
  FF_EN sw5/1 -> Add3/2
  FF_EN sw4/1 -> Add11/2
  Add11/1 -> Add3/1
  Gain3/1 -> Add10/2
  Gain2/1 -> Add10/1
  Add10/1 -> Integrator1/1
  Add8/1 -> Out4/1  "Dtot"
  In8/1 -> Add8/2  "Ddeg"
  In2/1 -> Add8/1  "Dprod"
  Gain7/1 -> Add6/1
  Add5/1 -> Out8/1  "rate_rv_tot"
  Add6/1 -> Add9/1, Add5/2, Gain3/1
  FF_EN sw2/1 -> Add9/2
  FF_EN sw3/1 -> Add5/1
  Gain4/1 -> Out6/1, FF_EN sw2/1, FF_EN sw3/1, FF_EN sw5/1  "rate_rv"
  Gain6/1 -> Out11/1  "Cfree_copy"
  Product2/1 -> Gain4/1
  In7/1 -> Gain5/1, Product2/2  "Dfree"
  In6/1 -> Gain7/1, Product2/1, Gain6/1  "Cfree"
  In5/1 -> Add6/2  "Cdeg"
  FF_EN sw1/1 -> Add7/1
  Manual Switch/1 -> Out1/1, A_FB_EN sw/1, B_FB_EN sw/1  "Ctot"
  Integrator1/1 -> Manual Switch/2
  In3/1 -> Manual Switch/1  "Ctot_in"
  Add9/1 -> Out10/1  "rate_rv_up"
  Add7/1 -> Out9/1  "rate_fw_up"
  FF_EN sw/1 -> Add4/2
  Add4/1 -> Out7/1  "rate_fw_tot"
  In4/1 -> Add7/2, Add4/1, Add11/1  "Cprod"
  Product1/1 -> FF_EN sw1/1, FF_EN sw4/1, FF_EN sw/1, Out5/1  "rate_fw"
  Exponential/1 -> Product1/2
  Gain1/1 -> Exponential/1
  In9/1 -> Add2/1  "Btot"
  In1/1 -> Add1/2  "Atot"
  Add1/1 -> Product1/1, Out2/1  "Afree"
  Add2/1 -> Out3/1, Gain1/1  "Bfree"
  Add3/1 -> Gain2/1
  A_FB_EN sw/1 -> Add1/1
  B_FB_EN sw/1 -> Add2/2
  Gain5/1 -> Out13/1  "Dfree_copy"

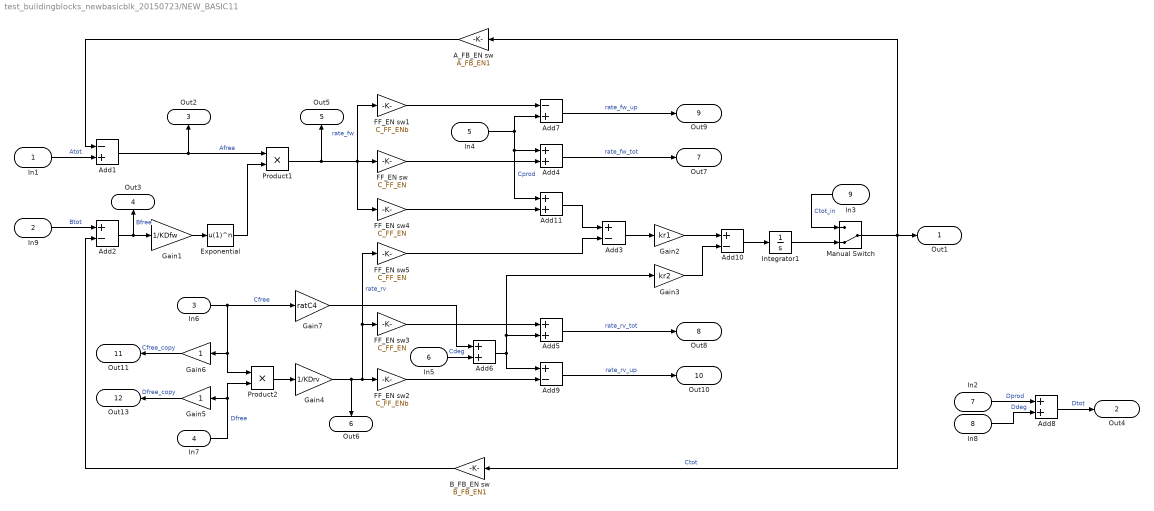
== system test_buildingblocks_newbasicblk_20150723/NEW_BASIC11 ==
  In1 : Inport
  In9 : Inport  Port=2
  In6 : Inport  Port=3
  In7 : Inport  Port=4
  In4 : Inport  Port=5
  In5 : Inport  Port=6
  In2 : Inport  Port=7
  In8 : Inport  Port=8
  In3 : Inport  Port=9
  A_FB_EN sw : Gain  Gain=A_FB_EN1
  Add1 : Sum  Inputs=-+
  Add{2..3,9..10} (4 alike) : Sum  Inputs=+-
  Add{4..6,8,11} (5 alike) : Sum
  Add7 : Sum  Inputs=-+
  B_FB_EN sw : Gain  Gain=B_FB_EN1
  Exponential : Fcn  Expr=u(1)^n
  FF_EN sw{,3..5} (4 alike) : Gain  Gain=C_FF_EN
  FF_EN sw1 : Gain  Gain=C_FF_ENb
  FF_EN sw2 : Gain  Gain=C_FF_ENb
  Gain1 : Gain  Gain=1/KDfw
  Gain2 : Gain  Gain=kr1
  Gain3 : Gain  Gain=kr2
  Gain4 : Gain  Gain=1/KDrv
  Gain5 : Gain
  Gain6 : Gain
  Gain7 : Gain  Gain=ratC4
  Integrator1 : Integrator
  Manual Switch : ManualSwitch  CurrentSetting=0
  Product1 : Product  RndMeth=Zero
  Product2 : Product  RndMeth=Zero
  Out1 : Outport
  Out4 : Outport  Port=2
  Out2 : Outport  Port=3
  Out3 : Outport  Port=4
  Out5 : Outport  Port=5
  Out6 : Outport  Port=6
  Out7 : Outport  Port=7
  Out8 : Outport  Port=8
  Out9 : Outport  Port=9
  Out10 : Outport  Port=10
  Out11 : Outport  Port=11
  Out13 : Outport  Port=12
  wires:
  Gain5/1 -> Out13/1  "Dfree_copy"
  B_FB_EN sw/1 -> Add2/2
  A_FB_EN sw/1 -> Add1/1
  Add3/1 -> Gain2/1
  Add2/1 -> Gain1/1, Out3/1  "Bfree"
  Add1/1 -> Out2/1, Product1/1  "Afree"
  In1/1 -> Add1/2  "Atot"
  In9/1 -> Add2/1  "Btot"
  Gain1/1 -> Exponential/1
  Exponential/1 -> Product1/2
  Product1/1 -> Out5/1, FF_EN sw/1, FF_EN sw4/1, FF_EN sw1/1  "rate_fw"
  In4/1 -> Add11/1, Add4/1, Add7/2  "Cprod"
  Add4/1 -> Out7/1  "rate_fw_tot"
  FF_EN sw/1 -> Add4/2
  Add7/1 -> Out9/1  "rate_fw_up"
  Add9/1 -> Out10/1  "rate_rv_up"
  In3/1 -> Manual Switch/1  "Ctot_in"
  Integrator1/1 -> Manual Switch/2
  Manual Switch/1 -> B_FB_EN sw/1, A_FB_EN sw/1, Out1/1  "Ctot"
  FF_EN sw1/1 -> Add7/1
  In5/1 -> Add6/2  "Cdeg"
  In6/1 -> Gain6/1, Product2/1, Gain7/1  "Cfree"
  In7/1 -> Product2/2, Gain5/1  "Dfree"
  Product2/1 -> Gain4/1
  Gain6/1 -> Out11/1  "Cfree_copy"
  Gain4/1 -> FF_EN sw5/1, FF_EN sw3/1, FF_EN sw2/1, Out6/1  "rate_rv"
  FF_EN sw3/1 -> Add5/1
  FF_EN sw2/1 -> Add9/2
  Add6/1 -> Gain3/1, Add5/2, Add9/1
  Add5/1 -> Out8/1  "rate_rv_tot"
  Gain7/1 -> Add6/1
  In2/1 -> Add8/1  "Dprod"
  In8/1 -> Add8/2  "Ddeg"
  Add8/1 -> Out4/1  "Dtot"
  Add10/1 -> Integrator1/1
  Gain2/1 -> Add10/1
  Gain3/1 -> Add10/2
  Add11/1 -> Add3/1
  FF_EN sw4/1 -> Add11/2
  FF_EN sw5/1 -> Add3/2

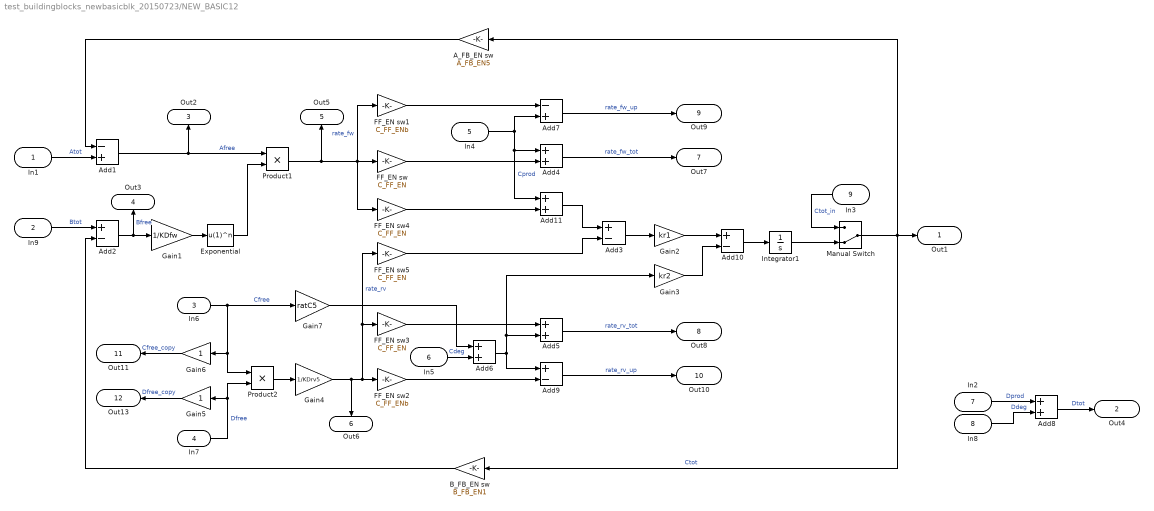
== system test_buildingblocks_newbasicblk_20150723/NEW_BASIC12 ==
  In1 : Inport
  In9 : Inport  Port=2
  In6 : Inport  Port=3
  In7 : Inport  Port=4
  In4 : Inport  Port=5
  In5 : Inport  Port=6
  In2 : Inport  Port=7
  In8 : Inport  Port=8
  In3 : Inport  Port=9
  A_FB_EN sw : Gain  Gain=A_FB_EN5
  Add1 : Sum  Inputs=-+
  Add{2..3,9..10} (4 alike) : Sum  Inputs=+-
  Add{4..6,8,11} (5 alike) : Sum
  Add7 : Sum  Inputs=-+
  B_FB_EN sw : Gain  Gain=B_FB_EN1
  Exponential : Fcn  Expr=u(1)^n
  FF_EN sw{,3..5} (4 alike) : Gain  Gain=C_FF_EN
  FF_EN sw1 : Gain  Gain=C_FF_ENb
  FF_EN sw2 : Gain  Gain=C_FF_ENb
  Gain1 : Gain  Gain=1/KDfw
  Gain2 : Gain  Gain=kr1
  Gain3 : Gain  Gain=kr2
  Gain4 : Gain  Gain=1/KDrv5
  Gain5 : Gain
  Gain6 : Gain
  Gain7 : Gain  Gain=ratC5
  Integrator1 : Integrator
  Manual Switch : ManualSwitch  CurrentSetting=0
  Product1 : Product  RndMeth=Zero
  Product2 : Product  RndMeth=Zero
  Out1 : Outport
  Out4 : Outport  Port=2
  Out2 : Outport  Port=3
  Out3 : Outport  Port=4
  Out5 : Outport  Port=5
  Out6 : Outport  Port=6
  Out7 : Outport  Port=7
  Out8 : Outport  Port=8
  Out9 : Outport  Port=9
  Out10 : Outport  Port=10
  Out11 : Outport  Port=11
  Out13 : Outport  Port=12
  wires:
  FF_EN sw5/1 -> Add3/2
  FF_EN sw4/1 -> Add11/2
  Add11/1 -> Add3/1
  Gain3/1 -> Add10/2
  Gain2/1 -> Add10/1
  Add10/1 -> Integrator1/1
  Add8/1 -> Out4/1  "Dtot"
  In8/1 -> Add8/2  "Ddeg"
  In2/1 -> Add8/1  "Dprod"
  Gain7/1 -> Add6/1
  Add5/1 -> Out8/1  "rate_rv_tot"
  Add6/1 -> Add9/1, Add5/2, Gain3/1
  FF_EN sw2/1 -> Add9/2
  FF_EN sw3/1 -> Add5/1
  Gain4/1 -> Out6/1, FF_EN sw2/1, FF_EN sw3/1, FF_EN sw5/1  "rate_rv"
  Gain6/1 -> Out11/1  "Cfree_copy"
  Product2/1 -> Gain4/1
  In7/1 -> Gain5/1, Product2/2  "Dfree"
  In6/1 -> Gain7/1, Product2/1, Gain6/1  "Cfree"
  In5/1 -> Add6/2  "Cdeg"
  FF_EN sw1/1 -> Add7/1
  Manual Switch/1 -> Out1/1, A_FB_EN sw/1, B_FB_EN sw/1  "Ctot"
  Integrator1/1 -> Manual Switch/2
  In3/1 -> Manual Switch/1  "Ctot_in"
  Add9/1 -> Out10/1  "rate_rv_up"
  Add7/1 -> Out9/1  "rate_fw_up"
  FF_EN sw/1 -> Add4/2
  Add4/1 -> Out7/1  "rate_fw_tot"
  In4/1 -> Add7/2, Add4/1, Add11/1  "Cprod"
  Product1/1 -> FF_EN sw1/1, FF_EN sw4/1, FF_EN sw/1, Out5/1  "rate_fw"
  Exponential/1 -> Product1/2
  Gain1/1 -> Exponential/1
  In9/1 -> Add2/1  "Btot"
  In1/1 -> Add1/2  "Atot"
  Add1/1 -> Product1/1, Out2/1  "Afree"
  Add2/1 -> Out3/1, Gain1/1  "Bfree"
  Add3/1 -> Gain2/1
  A_FB_EN sw/1 -> Add1/1
  B_FB_EN sw/1 -> Add2/2
  Gain5/1 -> Out13/1  "Dfree_copy"

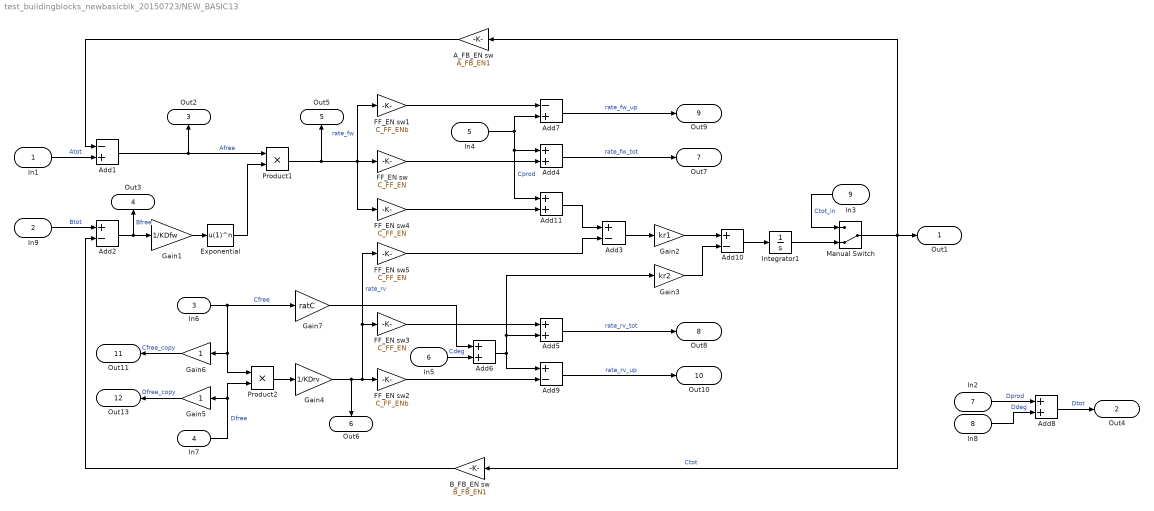
== system test_buildingblocks_newbasicblk_20150723/NEW_BASIC13 ==
  In1 : Inport
  In9 : Inport  Port=2
  In6 : Inport  Port=3
  In7 : Inport  Port=4
  In4 : Inport  Port=5
  In5 : Inport  Port=6
  In2 : Inport  Port=7
  In8 : Inport  Port=8
  In3 : Inport  Port=9
  A_FB_EN sw : Gain  Gain=A_FB_EN1
  Add1 : Sum  Inputs=-+
  Add{2..3,9..10} (4 alike) : Sum  Inputs=+-
  Add{4..6,8,11} (5 alike) : Sum
  Add7 : Sum  Inputs=-+
  B_FB_EN sw : Gain  Gain=B_FB_EN1
  Exponential : Fcn  Expr=u(1)^n
  FF_EN sw{,3..5} (4 alike) : Gain  Gain=C_FF_EN
  FF_EN sw1 : Gain  Gain=C_FF_ENb
  FF_EN sw2 : Gain  Gain=C_FF_ENb
  Gain1 : Gain  Gain=1/KDfw
  Gain2 : Gain  Gain=kr1
  Gain3 : Gain  Gain=kr2
  Gain4 : Gain  Gain=1/KDrv
  Gain5 : Gain
  Gain6 : Gain
  Gain7 : Gain  Gain=ratC
  Integrator1 : Integrator
  Manual Switch : ManualSwitch  CurrentSetting=0
  Product1 : Product  RndMeth=Zero
  Product2 : Product  RndMeth=Zero
  Out1 : Outport
  Out4 : Outport  Port=2
  Out2 : Outport  Port=3
  Out3 : Outport  Port=4
  Out5 : Outport  Port=5
  Out6 : Outport  Port=6
  Out7 : Outport  Port=7
  Out8 : Outport  Port=8
  Out9 : Outport  Port=9
  Out10 : Outport  Port=10
  Out11 : Outport  Port=11
  Out13 : Outport  Port=12
  wires:
  FF_EN sw5/1 -> Add3/2
  FF_EN sw4/1 -> Add11/2
  Add11/1 -> Add3/1
  Gain3/1 -> Add10/2
  Gain2/1 -> Add10/1
  Add10/1 -> Integrator1/1
  Add8/1 -> Out4/1  "Dtot"
  In8/1 -> Add8/2  "Ddeg"
  In2/1 -> Add8/1  "Dprod"
  Gain7/1 -> Add6/1
  Add5/1 -> Out8/1  "rate_rv_tot"
  Add6/1 -> Add9/1, Add5/2, Gain3/1
  FF_EN sw2/1 -> Add9/2
  FF_EN sw3/1 -> Add5/1
  Gain4/1 -> Out6/1, FF_EN sw2/1, FF_EN sw3/1, FF_EN sw5/1  "rate_rv"
  Gain6/1 -> Out11/1  "Cfree_copy"
  Product2/1 -> Gain4/1
  In7/1 -> Gain5/1, Product2/2  "Dfree"
  In6/1 -> Gain7/1, Product2/1, Gain6/1  "Cfree"
  In5/1 -> Add6/2  "Cdeg"
  FF_EN sw1/1 -> Add7/1
  Manual Switch/1 -> Out1/1, A_FB_EN sw/1, B_FB_EN sw/1  "Ctot"
  Integrator1/1 -> Manual Switch/2
  In3/1 -> Manual Switch/1  "Ctot_in"
  Add9/1 -> Out10/1  "rate_rv_up"
  Add7/1 -> Out9/1  "rate_fw_up"
  FF_EN sw/1 -> Add4/2
  Add4/1 -> Out7/1  "rate_fw_tot"
  In4/1 -> Add7/2, Add4/1, Add11/1  "Cprod"
  Product1/1 -> FF_EN sw1/1, FF_EN sw4/1, FF_EN sw/1, Out5/1  "rate_fw"
  Exponential/1 -> Product1/2
  Gain1/1 -> Exponential/1
  In9/1 -> Add2/1  "Btot"
  In1/1 -> Add1/2  "Atot"
  Add1/1 -> Product1/1, Out2/1  "Afree"
  Add2/1 -> Out3/1, Gain1/1  "Bfree"
  Add3/1 -> Gain2/1
  A_FB_EN sw/1 -> Add1/1
  B_FB_EN sw/1 -> Add2/2
  Gain5/1 -> Out13/1  "Dfree_copy"

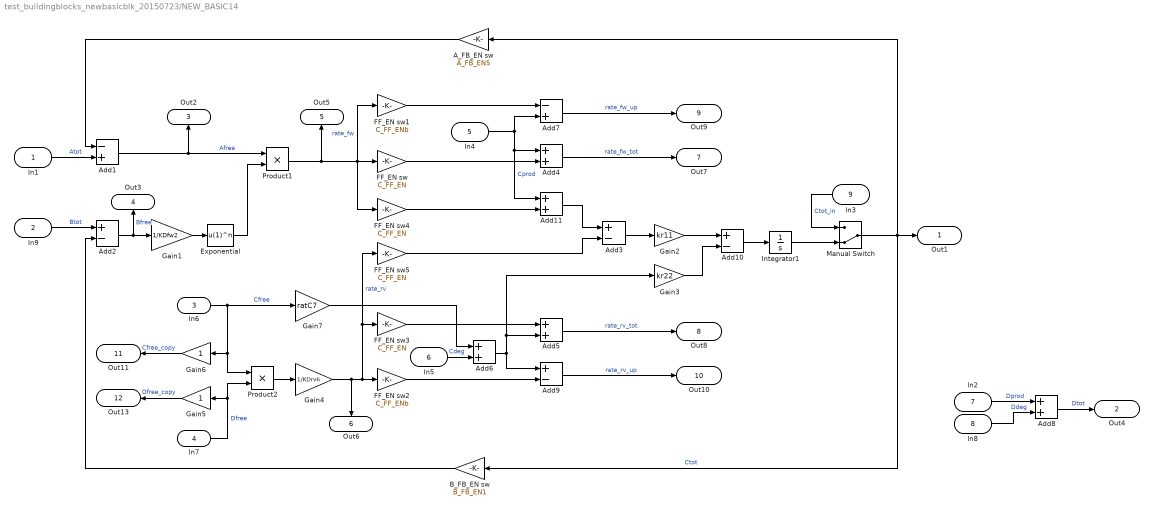
== system test_buildingblocks_newbasicblk_20150723/NEW_BASIC14 ==
  In1 : Inport
  In9 : Inport  Port=2
  In6 : Inport  Port=3
  In7 : Inport  Port=4
  In4 : Inport  Port=5
  In5 : Inport  Port=6
  In2 : Inport  Port=7
  In8 : Inport  Port=8
  In3 : Inport  Port=9
  A_FB_EN sw : Gain  Gain=A_FB_EN5
  Add1 : Sum  Inputs=-+
  Add{2..3,9..10} (4 alike) : Sum  Inputs=+-
  Add{4..6,8,11} (5 alike) : Sum
  Add7 : Sum  Inputs=-+
  B_FB_EN sw : Gain  Gain=B_FB_EN1
  Exponential : Fcn  Expr=u(1)^n
  FF_EN sw{,3..5} (4 alike) : Gain  Gain=C_FF_EN
  FF_EN sw1 : Gain  Gain=C_FF_ENb
  FF_EN sw2 : Gain  Gain=C_FF_ENb
  Gain1 : Gain  Gain=1/KDfw2
  Gain2 : Gain  Gain=kr11
  Gain3 : Gain  Gain=kr22
  Gain4 : Gain  Gain=1/KDrv6
  Gain5 : Gain
  Gain6 : Gain
  Gain7 : Gain  Gain=ratC7
  Integrator1 : Integrator
  Manual Switch : ManualSwitch  CurrentSetting=0
  Product1 : Product  RndMeth=Zero
  Product2 : Product  RndMeth=Zero
  Out1 : Outport
  Out4 : Outport  Port=2
  Out2 : Outport  Port=3
  Out3 : Outport  Port=4
  Out5 : Outport  Port=5
  Out6 : Outport  Port=6
  Out7 : Outport  Port=7
  Out8 : Outport  Port=8
  Out9 : Outport  Port=9
  Out10 : Outport  Port=10
  Out11 : Outport  Port=11
  Out13 : Outport  Port=12
  wires:
  Gain5/1 -> Out13/1  "Dfree_copy"
  B_FB_EN sw/1 -> Add2/2
  A_FB_EN sw/1 -> Add1/1
  Add3/1 -> Gain2/1
  Add2/1 -> Gain1/1, Out3/1  "Bfree"
  Add1/1 -> Out2/1, Product1/1  "Afree"
  In1/1 -> Add1/2  "Atot"
  In9/1 -> Add2/1  "Btot"
  Gain1/1 -> Exponential/1
  Exponential/1 -> Product1/2
  Product1/1 -> Out5/1, FF_EN sw/1, FF_EN sw4/1, FF_EN sw1/1  "rate_fw"
  In4/1 -> Add11/1, Add4/1, Add7/2  "Cprod"
  Add4/1 -> Out7/1  "rate_fw_tot"
  FF_EN sw/1 -> Add4/2
  Add7/1 -> Out9/1  "rate_fw_up"
  Add9/1 -> Out10/1  "rate_rv_up"
  In3/1 -> Manual Switch/1  "Ctot_in"
  Integrator1/1 -> Manual Switch/2
  Manual Switch/1 -> B_FB_EN sw/1, A_FB_EN sw/1, Out1/1  "Ctot"
  FF_EN sw1/1 -> Add7/1
  In5/1 -> Add6/2  "Cdeg"
  In6/1 -> Gain6/1, Product2/1, Gain7/1  "Cfree"
  In7/1 -> Product2/2, Gain5/1  "Dfree"
  Product2/1 -> Gain4/1
  Gain6/1 -> Out11/1  "Cfree_copy"
  Gain4/1 -> FF_EN sw5/1, FF_EN sw3/1, FF_EN sw2/1, Out6/1  "rate_rv"
  FF_EN sw3/1 -> Add5/1
  FF_EN sw2/1 -> Add9/2
  Add6/1 -> Gain3/1, Add5/2, Add9/1
  Add5/1 -> Out8/1  "rate_rv_tot"
  Gain7/1 -> Add6/1
  In2/1 -> Add8/1  "Dprod"
  In8/1 -> Add8/2  "Ddeg"
  Add8/1 -> Out4/1  "Dtot"
  Add10/1 -> Integrator1/1
  Gain2/1 -> Add10/1
  Gain3/1 -> Add10/2
  Add11/1 -> Add3/1
  FF_EN sw4/1 -> Add11/2
  FF_EN sw5/1 -> Add3/2

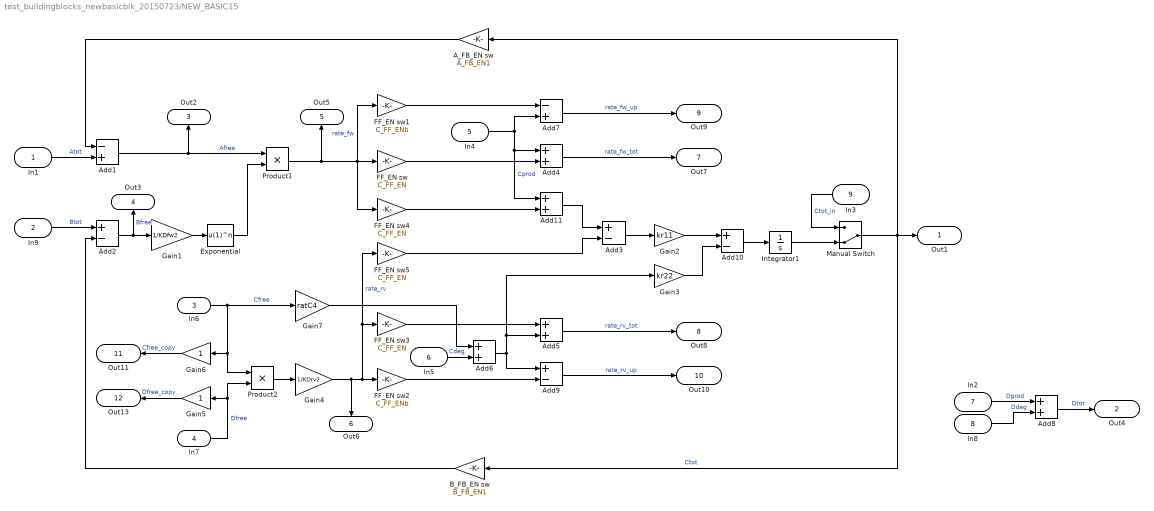
== system test_buildingblocks_newbasicblk_20150723/NEW_BASIC15 ==
  In1 : Inport
  In9 : Inport  Port=2
  In6 : Inport  Port=3
  In7 : Inport  Port=4
  In4 : Inport  Port=5
  In5 : Inport  Port=6
  In2 : Inport  Port=7
  In8 : Inport  Port=8
  In3 : Inport  Port=9
  A_FB_EN sw : Gain  Gain=A_FB_EN1
  Add1 : Sum  Inputs=-+
  Add{2..3,9..10} (4 alike) : Sum  Inputs=+-
  Add{4..6,8,11} (5 alike) : Sum
  Add7 : Sum  Inputs=-+
  B_FB_EN sw : Gain  Gain=B_FB_EN1
  Exponential : Fcn  Expr=u(1)^n
  FF_EN sw{,3..5} (4 alike) : Gain  Gain=C_FF_EN
  FF_EN sw1 : Gain  Gain=C_FF_ENb
  FF_EN sw2 : Gain  Gain=C_FF_ENb
  Gain1 : Gain  Gain=1/KDfw2
  Gain2 : Gain  Gain=kr11
  Gain3 : Gain  Gain=kr22
  Gain4 : Gain  Gain=1/KDrv2
  Gain5 : Gain
  Gain6 : Gain
  Gain7 : Gain  Gain=ratC4
  Integrator1 : Integrator
  Manual Switch : ManualSwitch  CurrentSetting=0
  Product1 : Product  RndMeth=Zero
  Product2 : Product  RndMeth=Zero
  Out1 : Outport
  Out4 : Outport  Port=2
  Out2 : Outport  Port=3
  Out3 : Outport  Port=4
  Out5 : Outport  Port=5
  Out6 : Outport  Port=6
  Out7 : Outport  Port=7
  Out8 : Outport  Port=8
  Out9 : Outport  Port=9
  Out10 : Outport  Port=10
  Out11 : Outport  Port=11
  Out13 : Outport  Port=12
  wires:
  FF_EN sw5/1 -> Add3/2
  FF_EN sw4/1 -> Add11/2
  Add11/1 -> Add3/1
  Gain3/1 -> Add10/2
  Gain2/1 -> Add10/1
  Add10/1 -> Integrator1/1
  Add8/1 -> Out4/1  "Dtot"
  In8/1 -> Add8/2  "Ddeg"
  In2/1 -> Add8/1  "Dprod"
  Gain7/1 -> Add6/1
  Add5/1 -> Out8/1  "rate_rv_tot"
  Add6/1 -> Add9/1, Add5/2, Gain3/1
  FF_EN sw2/1 -> Add9/2
  FF_EN sw3/1 -> Add5/1
  Gain4/1 -> Out6/1, FF_EN sw2/1, FF_EN sw3/1, FF_EN sw5/1  "rate_rv"
  Gain6/1 -> Out11/1  "Cfree_copy"
  Product2/1 -> Gain4/1
  In7/1 -> Gain5/1, Product2/2  "Dfree"
  In6/1 -> Gain7/1, Product2/1, Gain6/1  "Cfree"
  In5/1 -> Add6/2  "Cdeg"
  FF_EN sw1/1 -> Add7/1
  Manual Switch/1 -> Out1/1, A_FB_EN sw/1, B_FB_EN sw/1  "Ctot"
  Integrator1/1 -> Manual Switch/2
  In3/1 -> Manual Switch/1  "Ctot_in"
  Add9/1 -> Out10/1  "rate_rv_up"
  Add7/1 -> Out9/1  "rate_fw_up"
  FF_EN sw/1 -> Add4/2
  Add4/1 -> Out7/1  "rate_fw_tot"
  In4/1 -> Add7/2, Add4/1, Add11/1  "Cprod"
  Product1/1 -> FF_EN sw1/1, FF_EN sw4/1, FF_EN sw/1, Out5/1  "rate_fw"
  Exponential/1 -> Product1/2
  Gain1/1 -> Exponential/1
  In9/1 -> Add2/1  "Btot"
  In1/1 -> Add1/2  "Atot"
  Add1/1 -> Product1/1, Out2/1  "Afree"
  Add2/1 -> Out3/1, Gain1/1  "Bfree"
  Add3/1 -> Gain2/1
  A_FB_EN sw/1 -> Add1/1
  B_FB_EN sw/1 -> Add2/2
  Gain5/1 -> Out13/1  "Dfree_copy"

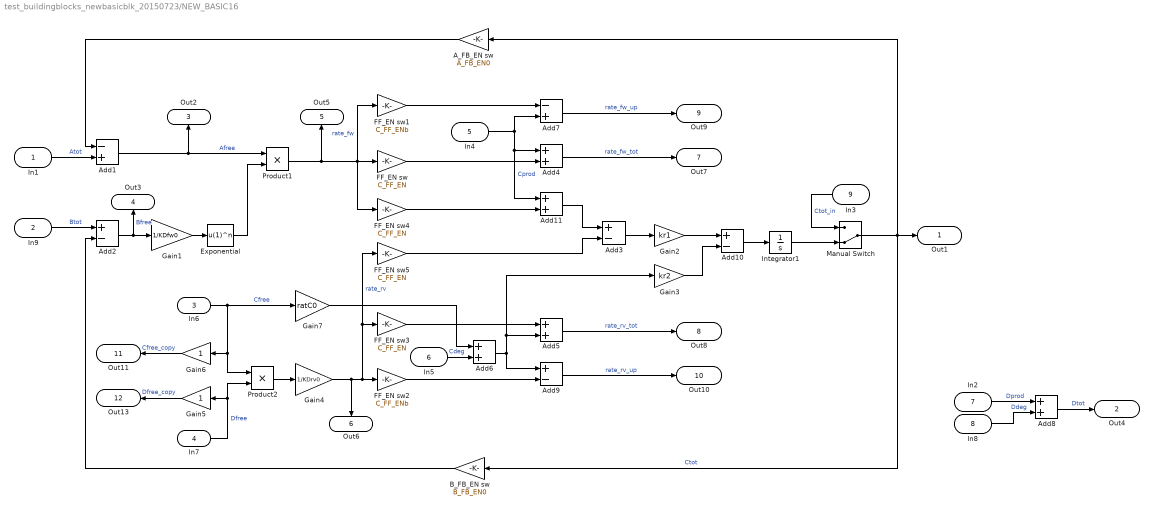
== system test_buildingblocks_newbasicblk_20150723/NEW_BASIC16 ==
  In1 : Inport
  In9 : Inport  Port=2
  In6 : Inport  Port=3
  In7 : Inport  Port=4
  In4 : Inport  Port=5
  In5 : Inport  Port=6
  In2 : Inport  Port=7
  In8 : Inport  Port=8
  In3 : Inport  Port=9
  A_FB_EN sw : Gain  Gain=A_FB_EN0
  Add1 : Sum  Inputs=-+
  Add{2..3,9..10} (4 alike) : Sum  Inputs=+-
  Add{4..6,8,11} (5 alike) : Sum
  Add7 : Sum  Inputs=-+
  B_FB_EN sw : Gain  Gain=B_FB_EN0
  Exponential : Fcn  Expr=u(1)^n
  FF_EN sw{,3..5} (4 alike) : Gain  Gain=C_FF_EN
  FF_EN sw1 : Gain  Gain=C_FF_ENb
  FF_EN sw2 : Gain  Gain=C_FF_ENb
  Gain1 : Gain  Gain=1/KDfw0
  Gain2 : Gain  Gain=kr1
  Gain3 : Gain  Gain=kr2
  Gain4 : Gain  Gain=1/KDrv0
  Gain5 : Gain
  Gain6 : Gain
  Gain7 : Gain  Gain=ratC0
  Integrator1 : Integrator
  Manual Switch : ManualSwitch  CurrentSetting=0
  Product1 : Product  RndMeth=Zero
  Product2 : Product  RndMeth=Zero
  Out1 : Outport
  Out4 : Outport  Port=2
  Out2 : Outport  Port=3
  Out3 : Outport  Port=4
  Out5 : Outport  Port=5
  Out6 : Outport  Port=6
  Out7 : Outport  Port=7
  Out8 : Outport  Port=8
  Out9 : Outport  Port=9
  Out10 : Outport  Port=10
  Out11 : Outport  Port=11
  Out13 : Outport  Port=12
  wires:
  Gain5/1 -> Out13/1  "Dfree_copy"
  B_FB_EN sw/1 -> Add2/2
  A_FB_EN sw/1 -> Add1/1
  Add3/1 -> Gain2/1
  Add2/1 -> Gain1/1, Out3/1  "Bfree"
  Add1/1 -> Out2/1, Product1/1  "Afree"
  In1/1 -> Add1/2  "Atot"
  In9/1 -> Add2/1  "Btot"
  Gain1/1 -> Exponential/1
  Exponential/1 -> Product1/2
  Product1/1 -> Out5/1, FF_EN sw/1, FF_EN sw4/1, FF_EN sw1/1  "rate_fw"
  In4/1 -> Add11/1, Add4/1, Add7/2  "Cprod"
  Add4/1 -> Out7/1  "rate_fw_tot"
  FF_EN sw/1 -> Add4/2
  Add7/1 -> Out9/1  "rate_fw_up"
  Add9/1 -> Out10/1  "rate_rv_up"
  In3/1 -> Manual Switch/1  "Ctot_in"
  Integrator1/1 -> Manual Switch/2
  Manual Switch/1 -> B_FB_EN sw/1, A_FB_EN sw/1, Out1/1  "Ctot"
  FF_EN sw1/1 -> Add7/1
  In5/1 -> Add6/2  "Cdeg"
  In6/1 -> Gain6/1, Product2/1, Gain7/1  "Cfree"
  In7/1 -> Product2/2, Gain5/1  "Dfree"
  Product2/1 -> Gain4/1
  Gain6/1 -> Out11/1  "Cfree_copy"
  Gain4/1 -> FF_EN sw5/1, FF_EN sw3/1, FF_EN sw2/1, Out6/1  "rate_rv"
  FF_EN sw3/1 -> Add5/1
  FF_EN sw2/1 -> Add9/2
  Add6/1 -> Gain3/1, Add5/2, Add9/1
  Add5/1 -> Out8/1  "rate_rv_tot"
  Gain7/1 -> Add6/1
  In2/1 -> Add8/1  "Dprod"
  In8/1 -> Add8/2  "Ddeg"
  Add8/1 -> Out4/1  "Dtot"
  Add10/1 -> Integrator1/1
  Gain2/1 -> Add10/1
  Gain3/1 -> Add10/2
  Add11/1 -> Add3/1
  FF_EN sw4/1 -> Add11/2
  FF_EN sw5/1 -> Add3/2

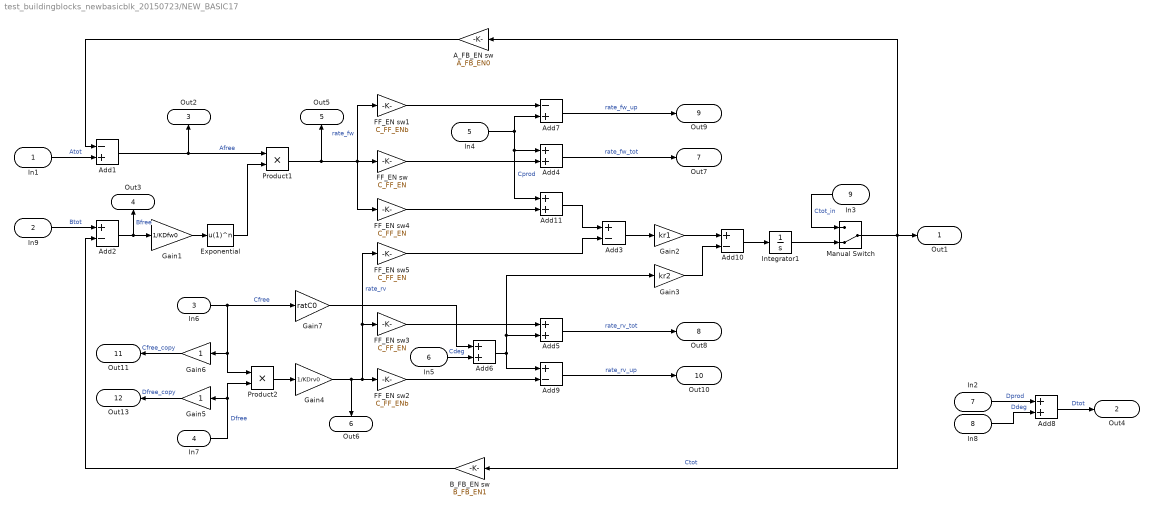
== system test_buildingblocks_newbasicblk_20150723/NEW_BASIC17 ==
  In1 : Inport
  In9 : Inport  Port=2
  In6 : Inport  Port=3
  In7 : Inport  Port=4
  In4 : Inport  Port=5
  In5 : Inport  Port=6
  In2 : Inport  Port=7
  In8 : Inport  Port=8
  In3 : Inport  Port=9
  A_FB_EN sw : Gain  Gain=A_FB_EN0
  Add1 : Sum  Inputs=-+
  Add{2..3,9..10} (4 alike) : Sum  Inputs=+-
  Add{4..6,8,11} (5 alike) : Sum
  Add7 : Sum  Inputs=-+
  B_FB_EN sw : Gain  Gain=B_FB_EN1
  Exponential : Fcn  Expr=u(1)^n
  FF_EN sw{,3..5} (4 alike) : Gain  Gain=C_FF_EN
  FF_EN sw1 : Gain  Gain=C_FF_ENb
  FF_EN sw2 : Gain  Gain=C_FF_ENb
  Gain1 : Gain  Gain=1/KDfw0
  Gain2 : Gain  Gain=kr1
  Gain3 : Gain  Gain=kr2
  Gain4 : Gain  Gain=1/KDrv0
  Gain5 : Gain
  Gain6 : Gain
  Gain7 : Gain  Gain=ratC0
  Integrator1 : Integrator
  Manual Switch : ManualSwitch  CurrentSetting=0
  Product1 : Product  RndMeth=Zero
  Product2 : Product  RndMeth=Zero
  Out1 : Outport
  Out4 : Outport  Port=2
  Out2 : Outport  Port=3
  Out3 : Outport  Port=4
  Out5 : Outport  Port=5
  Out6 : Outport  Port=6
  Out7 : Outport  Port=7
  Out8 : Outport  Port=8
  Out9 : Outport  Port=9
  Out10 : Outport  Port=10
  Out11 : Outport  Port=11
  Out13 : Outport  Port=12
  wires:
  Gain5/1 -> Out13/1  "Dfree_copy"
  B_FB_EN sw/1 -> Add2/2
  A_FB_EN sw/1 -> Add1/1
  Add3/1 -> Gain2/1
  Add2/1 -> Gain1/1, Out3/1  "Bfree"
  Add1/1 -> Out2/1, Product1/1  "Afree"
  In1/1 -> Add1/2  "Atot"
  In9/1 -> Add2/1  "Btot"
  Gain1/1 -> Exponential/1
  Exponential/1 -> Product1/2
  Product1/1 -> Out5/1, FF_EN sw/1, FF_EN sw4/1, FF_EN sw1/1  "rate_fw"
  In4/1 -> Add11/1, Add4/1, Add7/2  "Cprod"
  Add4/1 -> Out7/1  "rate_fw_tot"
  FF_EN sw/1 -> Add4/2
  Add7/1 -> Out9/1  "rate_fw_up"
  Add9/1 -> Out10/1  "rate_rv_up"
  In3/1 -> Manual Switch/1  "Ctot_in"
  Integrator1/1 -> Manual Switch/2
  Manual Switch/1 -> B_FB_EN sw/1, A_FB_EN sw/1, Out1/1  "Ctot"
  FF_EN sw1/1 -> Add7/1
  In5/1 -> Add6/2  "Cdeg"
  In6/1 -> Gain6/1, Product2/1, Gain7/1  "Cfree"
  In7/1 -> Product2/2, Gain5/1  "Dfree"
  Product2/1 -> Gain4/1
  Gain6/1 -> Out11/1  "Cfree_copy"
  Gain4/1 -> FF_EN sw5/1, FF_EN sw3/1, FF_EN sw2/1, Out6/1  "rate_rv"
  FF_EN sw3/1 -> Add5/1
  FF_EN sw2/1 -> Add9/2
  Add6/1 -> Gain3/1, Add5/2, Add9/1
  Add5/1 -> Out8/1  "rate_rv_tot"
  Gain7/1 -> Add6/1
  In2/1 -> Add8/1  "Dprod"
  In8/1 -> Add8/2  "Ddeg"
  Add8/1 -> Out4/1  "Dtot"
  Add10/1 -> Integrator1/1
  Gain2/1 -> Add10/1
  Gain3/1 -> Add10/2
  Add11/1 -> Add3/1
  FF_EN sw4/1 -> Add11/2
  FF_EN sw5/1 -> Add3/2
